simulink model "visRos2Comm"  (R2024b)
settings: Solver=VariableStepAuto  StartTime=0.0  StopTime=10.0  RelTol=1e-3
libraries: ros2lib x2
settings Model: Creator=Alyssa  LastModifiedBy=Alyssa

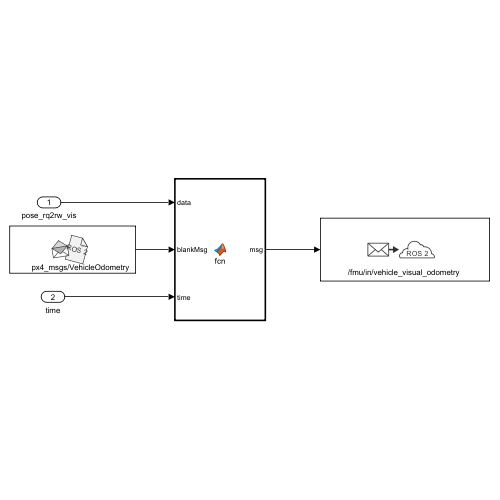
[thumbnail: Simulink's stored preview of the top-level diagram]
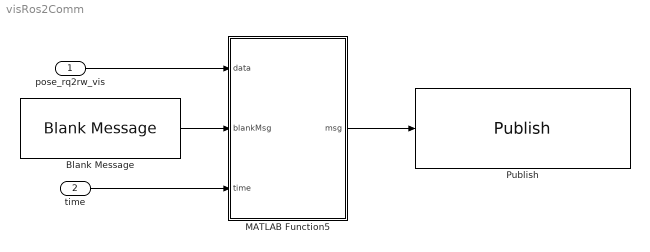
== system visRos2Comm ==
  pose_rq2rw_vis : Inport
  time : Inport  Port=2
  Blank Message : ros2lib/Blank Message  messageClass=Message  entityType=px4_msgs/VehicleOdometry  messageType=px4_msgs/VehicleOdometry  SampleTime=inf
  MATLAB Function5 : MATLAB Function  TreatAsAtomicUnit=on
  Publish : ros2lib/Publish  topicSource=Specify your own  topic=/fmu/in/vehicle_visual_odometry  messageType=px4_msgs/VehicleOdometry  QOSHistory=Keep last  QOSDepth=1  QOSReliability=Reliable  QOSDurability=Volatile  QOSDeadline=Inf  QOSLifespan=Inf  QOSLiveliness=Automatic  QOSLeaseDuration=Inf  QOSAvoidROSNamespaceConventions=off
  wires:
  MATLAB Function5/1(msg) -> Publish/1
  time/1 -> MATLAB Function5/3(time)
  pose_rq2rw_vis/1 -> MATLAB Function5/1(data)
  Blank Message/1 -> MATLAB Function5/2(blankMsg)

== matlab function visRos2Comm/MATLAB Function5 ==
  settings: updateMethod=DISCRETE  sampleTime=0.04
  data: data input; blankMsg input Bus: SL_Bus_px4_msgs_VehicleOdometry; msg output Bus: SL_Bus_px4_msgs_VehicleOdometry; time input
function msg = fcn(data, blankMsg, time)

%msg = ros2message("px4_msgs/VehicleOdometry");
msg = blankMsg;

%populate headers and other overhead info
timestamp_us = time * 1e6;
msg.timestamp = timestamp_us;
msg.timestamp_sample = timestamp_us;

msg.pose_frame = uint8(1); %set to POSE_FRAME_NED

msg.reset_counter = uint8(0);
msg.quality = int8(1);

%populate pose
%quat = tform2quat(data)';
%pos = tform2trvec(data)';
quat = data(4:7);
pos = data(1:3);

msg.position = single(pos);
msg.q = [single(quat(1)); single(quat(2)); single(quat(3)); single(quat(4))];

% %populate covariance - if all zeroes, px4 will reject
msg.position_variance = single([0.2; 0.2; 0.2]);
msg.orientation_variance = single([0.1; 0.1; 0.1]);

%disp('Sent pose');
